simulink model "magLev_GS_sim"  (R2016b)
settings: Solver=ode4  StartTime=0.0  StopTime=T  FixedStep=ts  RelTol=1e-3
values from neighbouring files (symbols this model uses):
  GainScheduling = Simulink.Parameter(GainScheduling)    [main.m]    (also in main_GS.m)
  sys = ss(A,B,C,D,      'name'     ,['Mag Lev trimmed p = ',num2str(position),' [m]'],      'StateName',{'p','v','i'},      'StateUnit',{'[m]','[m/s]','[A]'},      'InputName',{'V'},      'InputUnit',{'Volt'},      'OutputName',{'p'},      'OutputUnit',{'[m]'},      'UserData',trimPoint,      'Notes', [infoR,' | ',infoO])    [main.m]    (also in main_GS.m = ss(A,B,C,D,      'name'     ,['Mag Lev trimmed p = ',num2str)
  ts = 0.01    [main.m]    (also in main_GS.m)
  x0 = [2;0;0.2]    [main_GS.m]
settings Model: Creator=Gianni  LastModifiedBy=Gianni

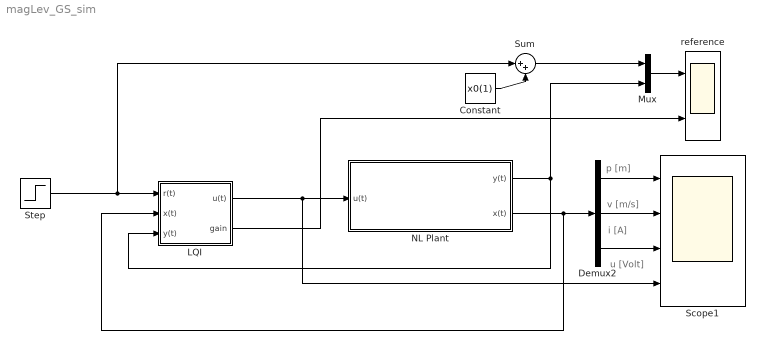
== system magLev_GS_sim ==
  note: u [Volt]
  note: i [A]
  note: v [m/s]
  note: p [m]
  Constant : Constant  Value=x0(1)
  Demux2 : Demux  Outputs=3
  LQI : Subsystem
  Mux : Mux  Inputs=2
  NL Plant : Subsystem
  Scope1 : Scope  NumInputPorts=4
  Step : Step  Time=5  Before=-1  SampleTime=0
  Sum : Sum  Inputs=|++
  reference : Scope  NumInputPorts=2
  wires:
  Demux2/1 -> Scope1/1
  Demux2/2 -> Scope1/2
  Demux2/3 -> Scope1/3
  NL Plant/1(y(t)) -> Mux/2, LQI/3(y(t))
  Mux/1 -> reference/1
  NL Plant/2(x(t)) -> LQI/2(x(t)), Demux2/1
  Step/1 -> Sum/1, LQI/1(r(t))
  LQI/1(u(t)) -> Scope1/4, NL Plant/1(u(t))
  Constant/1 -> Sum/2
  Sum/1 -> Mux/1
  LQI/2(gain) -> reference/2

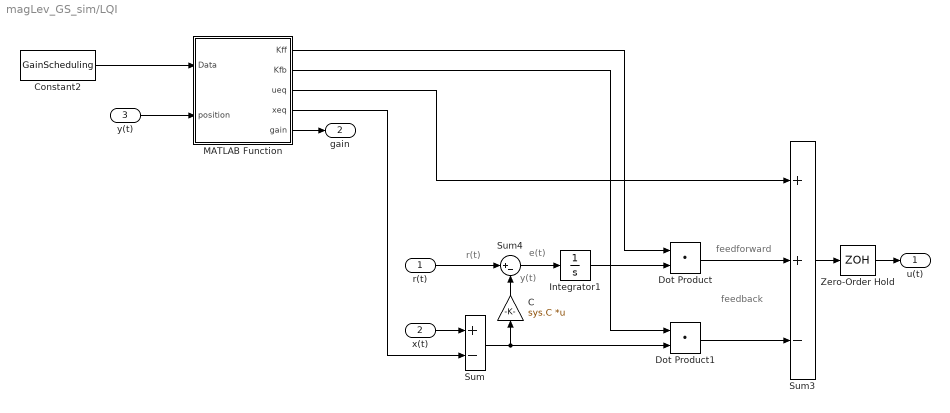
== system magLev_GS_sim/LQI ==
  note: feedforward
  note: feedback
  note: e(t)
  note: y(t)
  note: r(t)
  r(t) : Inport
  x(t) : Inport  Port=2
  y(t) : Inport  Port=3
  C : Gain  Gain=sys.C  Multiplication=Matrix(K*u)
  Constant2 : Constant  Value=GainScheduling  OutDataTypeStr=Bus: GainSchedulingStruct
  Dot Product : DotProduct  InputSameDT=on  OutDataTypeStr=Inherit: Inherit via internal rule
  Dot Product1 : DotProduct  InputSameDT=on  OutDataTypeStr=Inherit: Inherit via internal rule
  Integrator1 : Integrator
  MATLAB Function : MATLAB Function  TreatAsAtomicUnit=on
  Sum : Sum  Inputs=+-
  Sum3 : Sum  Inputs=++-
  Sum4 : Sum  Inputs=|+-
  Zero-Order Hold : ZeroOrderHold  SampleTime=ts
  u(t) : Outport
  gain : Outport  Port=2
  wires:
  C/1 -> Sum4/2
  Sum4/1 -> Integrator1/1
  Integrator1/1 -> Dot Product/2
  Sum3/1 -> Zero-Order Hold/1
  r(t)/1 -> Sum4/1
  x(t)/1 -> Sum/1
  Dot Product1/1 -> Sum3/3
  Constant2/1 -> MATLAB Function/1(Data)
  Dot Product/1 -> Sum3/2
  MATLAB Function/2(Kfb) -> Dot Product1/1
  MATLAB Function/3(ueq) -> Sum3/1
  MATLAB Function/1(Kff) -> Dot Product/1
  Sum/1 -> C/1, Dot Product1/2
  MATLAB Function/4(xeq) -> Sum/2
  Zero-Order Hold/1 -> u(t)/1
  y(t)/1 -> MATLAB Function/2(position)
  MATLAB Function/5(gain) -> gain/1

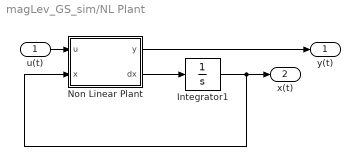
== system magLev_GS_sim/NL Plant ==
  u(t) : Inport
  Integrator1 : Integrator  InitialCondition=x0
  Non Linear Plant : MATLAB Function  TreatAsAtomicUnit=on
  y(t) : Outport
  x(t) : Outport  Port=2
  wires:
  u(t)/1 -> Non Linear Plant/1(u)
  Non Linear Plant/1(y) -> y(t)/1
  Integrator1/1 -> x(t)/1, Non Linear Plant/2(x)
  Non Linear Plant/2(dx) -> Integrator1/1

== matlab function magLev_GS_sim/LQI/MATLAB Function ==
  data: Data input; Kff output; Kfb output; ueq output; xeq output; position input; gain output
function [Kff,Kfb,ueq,xeq,gain] = fcn(Data,position)
    
    gain       = 1;               % initialize gain selector
    midpoint   = Data.GSmidpoint;   
    Ngain      = Data.Ngain;      % number of gains
    GSinterval = Data.GSinterval; % array with intervals 

    % select the gain;
    for i = 1:Ngain
        if (position >= GSinterval(i) && position < GSinterval(i+1))
            gain = i;     % parameter is withing GSinterval
        elseif (position < GSinterval(1))
            gain = 1;     % parameter is out the GSinterval (lower bound)
        elseif (position >= GSinterval(end))
            gain = Ngain; % parameter is out the GSinterval (upper bound)
        end
    end
    
    Kff = Data.Kff(:,gain);
    Kfb = Data.Kfb(:,gain);
    xeq = Data.xeq(:,midpoint);
    ueq = Data.ueq(:,midpoint);     
end

== matlab function magLev_GS_sim/NL Plant/Non Linear Plant ==
  data: u input; y output; x input; dx output
function [y,dx] = MagLev(u,x)

    g0 = 9.81;  R = 50;    L = 0.5;
    m  = 0.02; Km = 19.62; b = 0.1;
     
    x1 = x(1); % position [m]
    x2 = x(2); % velocity [m/s]
    x3 = x(3); % current  [A]

    %u % voltage  [V]

    dx = [x2;
          g0-(b/m)*x2-(Km/m)*((x3/x1)^2);
         (1/(L+Km/x1))*(-R*x3+Km*(x2/(x1^2))+u)];  
      y = x1;
end
